simulink model "ctrl_custom_case_c"  (R2016b)
settings: Solver=ode4  StartTime=0.0  StopTime=inf  FixedStep=0.01  RelTol=1e-3  EnableMultiTasking=on
undefined symbols (not defined in the file): alpha1, alpha2, b, C1, C2, center, D, inv_M, M, pd_final, pd_initial, R, Umax_1, Umax_2
libraries: lib x9, simulink x5
(part 3 of 3)

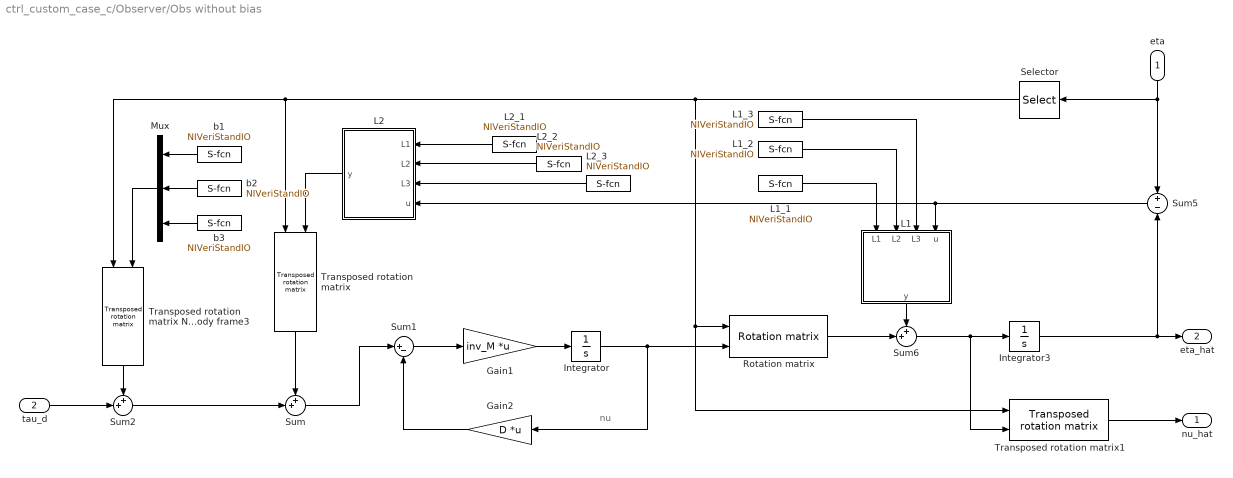
== system ctrl_custom_case_c/Observer/Obs without bias ==
  note: nu
  eta : Inport
  tau_d : Inport  Port=2
  Gain1 : Gain  Gain=inv_M  Multiplication=Matrix(K*u)
  Gain2 : Gain  Gain=D  Multiplication=Matrix(K*u)
  Integrator : Integrator
  Integrator3 : Integrator
  L1 : MATLAB Function  TreatAsAtomicUnit=on
  L1_1 : S-Function  Priority=1  FunctionName=NIVeriStandIO  Parameters=width dtype portnum stime stype btype  SFunctionDeploymentMode=off  EnableBusSupport=off  mask(NI VeriStand Inport){portnum=1, width=-1, stime=-1, dtype=auto, stype=auto, btype=1}
      mask prompts: portnum "Port number:"; width "Port dimensions (-1 for dynamically sized):"; stime "Sample time (-1 for inherited):"; dtype "Data type:"; stype "Signal type:"; btype "Block type:"
      mask help: Use this inport on any level of nested subsystems to allow NI VeriStand software to map signals to it.
      mask init:
      | NIVeriStandIO_init;
      settings: CopyFcn=NIVeriStand_MDL_functions('', 'IO_copy');  DeleteFcn=NIVeriStand_MDL_functions('', 'IO_delete');  MoveFcn=set_param(gcb, 'Mask', 'on');
      mask Callback portnum: NIVeriStand_MDL_functions('', 'IO_setportnum');
      mask TypeOptions dtype: auto | double | single | int8 | uint8 | int16 | uint16 | int32 | uint32 | boolean
      mask Callback dtype: NIVeriStand_MDL_functions('', 'IO_booleansignal');
      mask TypeOptions stype: auto | real | complex
      mask Display:
      | patch([-x x], [-y y], [.90980 .81960 .32156]);
      | plot([xrad -x x xrad], [yrad -y y yrad]);
      | fprintf('NI In%d', portnum);
  L1_2 : S-Function  Priority=2  FunctionName=NIVeriStandIO  Parameters=width dtype portnum stime stype btype  SFunctionDeploymentMode=off  EnableBusSupport=off  mask(NI VeriStand Inport){portnum=2, width=-1, stime=-1, dtype=auto, stype=auto, btype=1}
      mask prompts: portnum "Port number:"; width "Port dimensions (-1 for dynamically sized):"; stime "Sample time (-1 for inherited):"; dtype "Data type:"; stype "Signal type:"; btype "Block type:"
      mask help: Use this inport on any level of nested subsystems to allow NI VeriStand software to map signals to it.
      mask init:
      | NIVeriStandIO_init;
      settings: CopyFcn=NIVeriStand_MDL_functions('', 'IO_copy');  DeleteFcn=NIVeriStand_MDL_functions('', 'IO_delete');  MoveFcn=set_param(gcb, 'Mask', 'on');
      mask Callback portnum: NIVeriStand_MDL_functions('', 'IO_setportnum');
      mask TypeOptions dtype: auto | double | single | int8 | uint8 | int16 | uint16 | int32 | uint32 | boolean
      mask Callback dtype: NIVeriStand_MDL_functions('', 'IO_booleansignal');
      mask TypeOptions stype: auto | real | complex
      mask Display:
      | patch([-x x], [-y y], [.90980 .81960 .32156]);
      | plot([xrad -x x xrad], [yrad -y y yrad]);
      | fprintf('NI In%d', portnum);
  L1_3 : S-Function  Priority=3  FunctionName=NIVeriStandIO  Parameters=width dtype portnum stime stype btype  SFunctionDeploymentMode=off  EnableBusSupport=off  mask(NI VeriStand Inport){portnum=3, width=-1, stime=-1, dtype=auto, stype=auto, btype=1}
      mask prompts: portnum "Port number:"; width "Port dimensions (-1 for dynamically sized):"; stime "Sample time (-1 for inherited):"; dtype "Data type:"; stype "Signal type:"; btype "Block type:"
      mask help: Use this inport on any level of nested subsystems to allow NI VeriStand software to map signals to it.
      mask init:
      | NIVeriStandIO_init;
      settings: CopyFcn=NIVeriStand_MDL_functions('', 'IO_copy');  DeleteFcn=NIVeriStand_MDL_functions('', 'IO_delete');  MoveFcn=set_param(gcb, 'Mask', 'on');
      mask Callback portnum: NIVeriStand_MDL_functions('', 'IO_setportnum');
      mask TypeOptions dtype: auto | double | single | int8 | uint8 | int16 | uint16 | int32 | uint32 | boolean
      mask Callback dtype: NIVeriStand_MDL_functions('', 'IO_booleansignal');
      mask TypeOptions stype: auto | real | complex
      mask Display:
      | patch([-x x], [-y y], [.90980 .81960 .32156]);
      | plot([xrad -x x xrad], [yrad -y y yrad]);
      | fprintf('NI In%d', portnum);
  L2 : MATLAB Function  TreatAsAtomicUnit=on
  L2_1 : S-Function  Priority=4  FunctionName=NIVeriStandIO  Parameters=width dtype portnum stime stype btype  SFunctionDeploymentMode=off  EnableBusSupport=off  mask(NI VeriStand Inport){portnum=4, width=-1, stime=-1, dtype=auto, stype=auto, btype=1}
      mask prompts: portnum "Port number:"; width "Port dimensions (-1 for dynamically sized):"; stime "Sample time (-1 for inherited):"; dtype "Data type:"; stype "Signal type:"; btype "Block type:"
      mask help: Use this inport on any level of nested subsystems to allow NI VeriStand software to map signals to it.
      mask init:
      | NIVeriStandIO_init;
      settings: CopyFcn=NIVeriStand_MDL_functions('', 'IO_copy');  DeleteFcn=NIVeriStand_MDL_functions('', 'IO_delete');  MoveFcn=set_param(gcb, 'Mask', 'on');
      mask Callback portnum: NIVeriStand_MDL_functions('', 'IO_setportnum');
      mask TypeOptions dtype: auto | double | single | int8 | uint8 | int16 | uint16 | int32 | uint32 | boolean
      mask Callback dtype: NIVeriStand_MDL_functions('', 'IO_booleansignal');
      mask TypeOptions stype: auto | real | complex
      mask Display:
      | patch([-x x], [-y y], [.90980 .81960 .32156]);
      | plot([xrad -x x xrad], [yrad -y y yrad]);
      | fprintf('NI In%d', portnum);
  L2_2 : S-Function  Priority=5  FunctionName=NIVeriStandIO  Parameters=width dtype portnum stime stype btype  SFunctionDeploymentMode=off  EnableBusSupport=off  mask(NI VeriStand Inport){portnum=5, width=-1, stime=-1, dtype=auto, stype=auto, btype=1}
      mask prompts: portnum "Port number:"; width "Port dimensions (-1 for dynamically sized):"; stime "Sample time (-1 for inherited):"; dtype "Data type:"; stype "Signal type:"; btype "Block type:"
      mask help: Use this inport on any level of nested subsystems to allow NI VeriStand software to map signals to it.
      mask init:
      | NIVeriStandIO_init;
      settings: CopyFcn=NIVeriStand_MDL_functions('', 'IO_copy');  DeleteFcn=NIVeriStand_MDL_functions('', 'IO_delete');  MoveFcn=set_param(gcb, 'Mask', 'on');
      mask Callback portnum: NIVeriStand_MDL_functions('', 'IO_setportnum');
      mask TypeOptions dtype: auto | double | single | int8 | uint8 | int16 | uint16 | int32 | uint32 | boolean
      mask Callback dtype: NIVeriStand_MDL_functions('', 'IO_booleansignal');
      mask TypeOptions stype: auto | real | complex
      mask Display:
      | patch([-x x], [-y y], [.90980 .81960 .32156]);
      | plot([xrad -x x xrad], [yrad -y y yrad]);
      | fprintf('NI In%d', portnum);
  L2_3 : S-Function  Priority=6  FunctionName=NIVeriStandIO  Parameters=width dtype portnum stime stype btype  SFunctionDeploymentMode=off  EnableBusSupport=off  mask(NI VeriStand Inport){portnum=6, width=-1, stime=-1, dtype=auto, stype=auto, btype=1}
      mask prompts: portnum "Port number:"; width "Port dimensions (-1 for dynamically sized):"; stime "Sample time (-1 for inherited):"; dtype "Data type:"; stype "Signal type:"; btype "Block type:"
      mask help: Use this inport on any level of nested subsystems to allow NI VeriStand software to map signals to it.
      mask init:
      | NIVeriStandIO_init;
      settings: CopyFcn=NIVeriStand_MDL_functions('', 'IO_copy');  DeleteFcn=NIVeriStand_MDL_functions('', 'IO_delete');  MoveFcn=set_param(gcb, 'Mask', 'on');
      mask Callback portnum: NIVeriStand_MDL_functions('', 'IO_setportnum');
      mask TypeOptions dtype: auto | double | single | int8 | uint8 | int16 | uint16 | int32 | uint32 | boolean
      mask Callback dtype: NIVeriStand_MDL_functions('', 'IO_booleansignal');
      mask TypeOptions stype: auto | real | complex
      mask Display:
      | patch([-x x], [-y y], [.90980 .81960 .32156]);
      | plot([xrad -x x xrad], [yrad -y y yrad]);
      | fprintf('NI In%d', portnum);
  Mux : Mux  Inputs=3
  Rotation matrix : lib/Rotation matrix
  Selector : Selector  InputPortWidth=3  IndexOptions=Index vector (dialog)  Indices=[ 3]  OutputSizes=1
  Sum : Sum  Inputs=++|
  Sum1 : Sum  Inputs=|+-
  Sum2 : Sum  Inputs=++|
  Sum5 : Sum  Inputs=+|-
  Sum6 : Sum  Inputs=++|
  Transposed rotation matrix : lib/Transposed rotation matrix
  "Transposed rotation matrix NED -> Body frame3" : lib/Transposed rotation matrix
  Transposed rotation matrix1 : lib/Transposed rotation matrix
  b1 : S-Function  Priority=7  FunctionName=NIVeriStandIO  Parameters=width dtype portnum stime stype btype  SFunctionDeploymentMode=off  EnableBusSupport=off  mask(NI VeriStand Inport){portnum=7, width=-1, stime=-1, dtype=auto, stype=auto, btype=1}
      mask prompts: portnum "Port number:"; width "Port dimensions (-1 for dynamically sized):"; stime "Sample time (-1 for inherited):"; dtype "Data type:"; stype "Signal type:"; btype "Block type:"
      mask help: Use this inport on any level of nested subsystems to allow NI VeriStand software to map signals to it.
      mask init:
      | NIVeriStandIO_init;
      settings: CopyFcn=NIVeriStand_MDL_functions('', 'IO_copy');  DeleteFcn=NIVeriStand_MDL_functions('', 'IO_delete');  MoveFcn=set_param(gcb, 'Mask', 'on');
      mask Callback portnum: NIVeriStand_MDL_functions('', 'IO_setportnum');
      mask TypeOptions dtype: auto | double | single | int8 | uint8 | int16 | uint16 | int32 | uint32 | boolean
      mask Callback dtype: NIVeriStand_MDL_functions('', 'IO_booleansignal');
      mask TypeOptions stype: auto | real | complex
      mask Display:
      | patch([-x x], [-y y], [.90980 .81960 .32156]);
      | plot([xrad -x x xrad], [yrad -y y yrad]);
      | fprintf('NI In%d', portnum);
  b2 : S-Function  Priority=8  FunctionName=NIVeriStandIO  Parameters=width dtype portnum stime stype btype  SFunctionDeploymentMode=off  EnableBusSupport=off  mask(NI VeriStand Inport){portnum=8, width=-1, stime=-1, dtype=auto, stype=auto, btype=1}
      mask prompts: portnum "Port number:"; width "Port dimensions (-1 for dynamically sized):"; stime "Sample time (-1 for inherited):"; dtype "Data type:"; stype "Signal type:"; btype "Block type:"
      mask help: Use this inport on any level of nested subsystems to allow NI VeriStand software to map signals to it.
      mask init:
      | NIVeriStandIO_init;
      settings: CopyFcn=NIVeriStand_MDL_functions('', 'IO_copy');  DeleteFcn=NIVeriStand_MDL_functions('', 'IO_delete');  MoveFcn=set_param(gcb, 'Mask', 'on');
      mask Callback portnum: NIVeriStand_MDL_functions('', 'IO_setportnum');
      mask TypeOptions dtype: auto | double | single | int8 | uint8 | int16 | uint16 | int32 | uint32 | boolean
      mask Callback dtype: NIVeriStand_MDL_functions('', 'IO_booleansignal');
      mask TypeOptions stype: auto | real | complex
      mask Display:
      | patch([-x x], [-y y], [.90980 .81960 .32156]);
      | plot([xrad -x x xrad], [yrad -y y yrad]);
      | fprintf('NI In%d', portnum);
  b3 : S-Function  Priority=9  FunctionName=NIVeriStandIO  Parameters=width dtype portnum stime stype btype  SFunctionDeploymentMode=off  EnableBusSupport=off  mask(NI VeriStand Inport){portnum=9, width=-1, stime=-1, dtype=auto, stype=auto, btype=1}
      mask prompts: portnum "Port number:"; width "Port dimensions (-1 for dynamically sized):"; stime "Sample time (-1 for inherited):"; dtype "Data type:"; stype "Signal type:"; btype "Block type:"
      mask help: Use this inport on any level of nested subsystems to allow NI VeriStand software to map signals to it.
      mask init:
      | NIVeriStandIO_init;
      settings: CopyFcn=NIVeriStand_MDL_functions('', 'IO_copy');  DeleteFcn=NIVeriStand_MDL_functions('', 'IO_delete');  MoveFcn=set_param(gcb, 'Mask', 'on');
      mask Callback portnum: NIVeriStand_MDL_functions('', 'IO_setportnum');
      mask TypeOptions dtype: auto | double | single | int8 | uint8 | int16 | uint16 | int32 | uint32 | boolean
      mask Callback dtype: NIVeriStand_MDL_functions('', 'IO_booleansignal');
      mask TypeOptions stype: auto | real | complex
      mask Display:
      | patch([-x x], [-y y], [.90980 .81960 .32156]);
      | plot([xrad -x x xrad], [yrad -y y yrad]);
      | fprintf('NI In%d', portnum);
  nu_hat : Outport
  eta_hat : Outport  Port=2
  wires:
  Sum/1 -> Sum1/1
  Sum6/1 -> Transposed rotation matrix1/2, Integrator3/1
  Transposed rotation matrix1/1 -> nu_hat/1
  L1/1(y) -> Sum6/1
  Rotation matrix/1 -> Sum6/2
  Sum5/1 -> L1/4(u), L2/4(u)
  Gain1/1 -> Integrator/1
  Integrator3/1 -> Sum5/2, eta_hat/1
  L2/1(y) -> Transposed rotation matrix/2
  Transposed rotation matrix/1 -> Sum/1
  Sum1/1 -> Gain1/1
  eta/1 -> Selector/1, Sum5/1
  Gain2/1 -> Sum1/2
  Integrator/1 -> Gain2/1, Rotation matrix/2
  L1_1/1 -> L1/1(L1)
  L1_2/1 -> L1/2(L2)
  L1_3/1 -> L1/3(L3)
  L2_1/1 -> L2/1(L1)
  L2_2/1 -> L2/2(L2)
  L2_3/1 -> L2/3(L3)
  Selector/1 -> Transposed rotation matrix1/1, Rotation matrix/1, Transposed rotation matrix/1, "Transposed rotation matrix NED -> Body frame3"/1
  Mux/1 -> "Transposed rotation matrix NED -> Body frame3"/2
  b1/1 -> Mux/1
  b2/1 -> Mux/2
  b3/1 -> Mux/3
  tau_d/1 -> Sum2/2
  Sum2/1 -> Sum/2
  "Transposed rotation matrix NED -> Body frame3"/1 -> Sum2/1

== system ctrl_custom_case_c/Thrust Allocation-rec/VSP1 ==
  u_1x : Inport
  u_1y : Inport  Port=2
  Atan2 : Trigonometry  Operator=atan2
  Sqrt : Sqrt  SaturateOnIntegerOverflow=on
  Square : Math  Operator=square  SaturateOnIntegerOverflow=on
  Square1 : Math  Operator=square  SaturateOnIntegerOverflow=on
  Sum : Sum  Inputs=|++
  u_1 : Outport
  Alpha_1 : Outport  Port=2
  wires:
  u_1x/1 -> Atan2/2, Square/1
  u_1y/1 -> Square1/1, Atan2/1
  Square/1 -> Sum/1
  Square1/1 -> Sum/2
  Sum/1 -> Sqrt/1
  Sqrt/1 -> u_1/1
  Atan2/1 -> Alpha_1/1

== system ctrl_custom_case_c/Thrust Allocation-rec/VSP2 ==
  u_2x : Inport
  u_2y : Inport  Port=2
  Atan2 : Trigonometry  Operator=atan2
  Sqrt : Sqrt  SaturateOnIntegerOverflow=on
  Square : Math  Operator=square  SaturateOnIntegerOverflow=on
  Square1 : Math  Operator=square  SaturateOnIntegerOverflow=on
  Sum : Sum  Inputs=|++
  u_2 : Outport
  Alpha_2 : Outport  Port=2
  wires:
  Square/1 -> Sum/1
  Square1/1 -> Sum/2
  Sum/1 -> Sqrt/1
  Sqrt/1 -> u_2/1
  u_2x/1 -> Atan2/2, Square/1
  Atan2/1 -> Alpha_2/1
  u_2y/1 -> Atan2/1, Square1/1

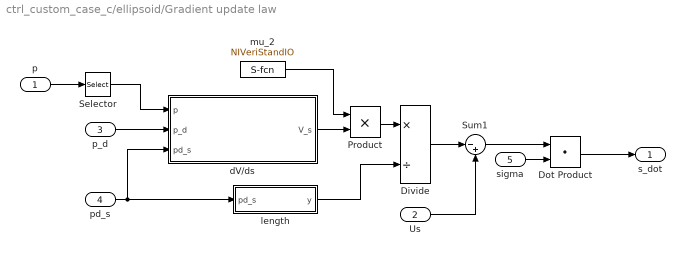
== system ctrl_custom_case_c/ellipsoid/Gradient update law ==
  p : Inport
  Us : Inport  Port=2
  p_d : Inport  Port=3
  pd_s : Inport  Port=4
  sigma : Inport  Port=5
  Divide : Product  Inputs=*/
  Dot Product : DotProduct  InputSameDT=on  OutDataTypeStr=Inherit: Inherit via internal rule
  Product : Product
  Selector : Selector  InputPortWidth=3  IndexOptions=Index vector (dialog)  Indices=[1 2]  OutputSizes=1
  Sum1 : Sum  Inputs=|-+
  "dV/ds  " : MATLAB Function  TreatAsAtomicUnit=on
  length : MATLAB Function  TreatAsAtomicUnit=on
  mu_2 : S-Function  Priority=1  FunctionName=NIVeriStandIO  Parameters=width dtype portnum stime stype btype  SFunctionDeploymentMode=off  EnableBusSupport=off  mask(NI VeriStand Inport){portnum=1, width=-1, stime=-1, dtype=auto, stype=auto, btype=1}
      mask prompts: portnum "Port number:"; width "Port dimensions (-1 for dynamically sized):"; stime "Sample time (-1 for inherited):"; dtype "Data type:"; stype "Signal type:"; btype "Block type:"
      mask help: Use this inport on any level of nested subsystems to allow NI VeriStand software to map signals to it.
      mask init:
      | NIVeriStandIO_init;
      settings: CopyFcn=NIVeriStand_MDL_functions('', 'IO_copy');  DeleteFcn=NIVeriStand_MDL_functions('', 'IO_delete');  MoveFcn=set_param(gcb, 'Mask', 'on');
      mask Callback portnum: NIVeriStand_MDL_functions('', 'IO_setportnum');
      mask TypeOptions dtype: auto | double | single | int8 | uint8 | int16 | uint16 | int32 | uint32 | boolean
      mask Callback dtype: NIVeriStand_MDL_functions('', 'IO_booleansignal');
      mask TypeOptions stype: auto | real | complex
      mask Display:
      | patch([-x x], [-y y], [.90980 .81960 .32156]);
      | plot([xrad -x x xrad], [yrad -y y yrad]);
      | fprintf('NI In%d', portnum);
  s_dot : Outport
  wires:
  Product/1 -> Divide/1
  Divide/1 -> Sum1/1
  "dV/ds  "/1(V_s) -> Product/2
  p_d/1 -> "dV/ds  "/2(p_d)
  pd_s/1 -> "dV/ds  "/3(pd_s), length/1(pd_s)
  length/1(y) -> Divide/2
  Us/1 -> Sum1/2
  Sum1/1 -> Dot Product/1
  Dot Product/1 -> s_dot/1
  sigma/1 -> Dot Product/2
  p/1 -> Selector/1
  Selector/1 -> "dV/ds  "/1(p)
  mu_2/1 -> Product/1

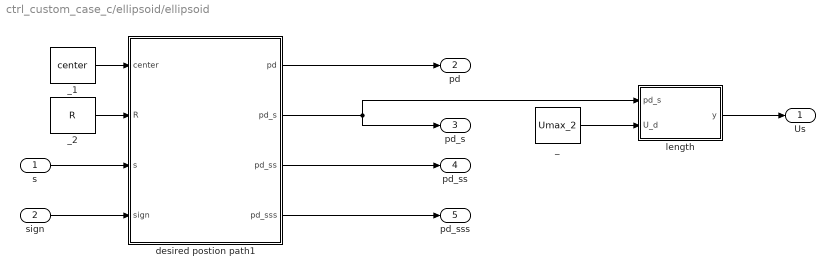
== system ctrl_custom_case_c/ellipsoid/ellipsoid ==
  s : Inport
  sign : Inport  Port=2
  _ : Constant  Value=Umax_2
  _1 : Constant  Value=center
  _2 : Constant  Value=R
  desired postion path1 : MATLAB Function  TreatAsAtomicUnit=on
  length : MATLAB Function  TreatAsAtomicUnit=on
  Us : Outport
  pd : Outport  Port=2
  pd_s : Outport  Port=3
  pd_ss : Outport  Port=4
  pd_sss : Outport  Port=5
  wires:
  _2/1 -> desired postion path1/2(R)
  _1/1 -> desired postion path1/1(center)
  desired postion path1/1(pd) -> pd/1
  desired postion path1/2(pd_s) -> pd_s/1, length/1(pd_s)
  length/1(y) -> Us/1
  s/1 -> desired postion path1/3(s)
  sign/1 -> desired postion path1/4(sign)
  _/1 -> length/2(U_d)
  desired postion path1/3(pd_ss) -> pd_ss/1
  desired postion path1/4(pd_sss) -> pd_sss/1

== system ctrl_custom_case_c/ellipsoid/position controller ==
  p : Inport
  pd : Inport  Port=2
  pd_s : Inport  Port=3
  Us : Inport  Port=4
  K : Gain  Gain=diag([0.1,0.1])  Multiplication=Matrix(K*u)
  Product : Product
  Selector : Selector  InputPortWidth=3  IndexOptions=Index vector (dialog)  Indices=[1 2]  OutputSizes=1
  Sum : Sum  Inputs=|+-
  Sum1 : Sum  Inputs=|-+
  u : Outport
  wires:
  Sum/1 -> K/1
  pd_s/1 -> Product/1
  Us/1 -> Product/2
  K/1 -> Sum1/1
  Product/1 -> Sum1/2
  Sum1/1 -> u/1
  pd/1 -> Sum/2
  p/1 -> Selector/1
  Selector/1 -> Sum/1

== system ctrl_custom_case_c/ellipsoid/switch ==
  s : Inport
  Memory : Memory  X0=1
  switch with respect to s : MATLAB Function  TreatAsAtomicUnit=on
  sign : Outport
  wires:
  switch with respect to s/1(sign_) -> sign/1, Memory/1
  Memory/1 -> switch with respect to s/2(prev_sign)
  s/1 -> switch with respect to s/1(s)

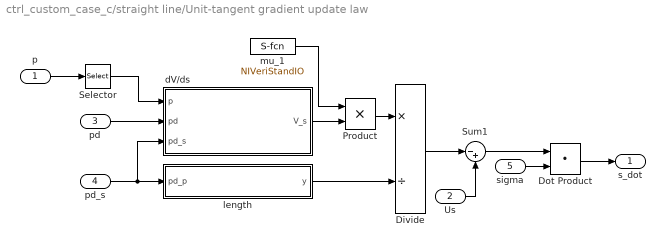
== system ctrl_custom_case_c/straight line/Unit-tangent gradient update law ==
  p : Inport
  Us : Inport  Port=2
  pd : Inport  Port=3
  pd_s : Inport  Port=4
  sigma : Inport  Port=5
  Divide : Product  Inputs=*/
  Dot Product : DotProduct  InputSameDT=on  OutDataTypeStr=Inherit: Inherit via internal rule
  Product : Product
  Selector : Selector  InputPortWidth=3  IndexOptions=Index vector (dialog)  Indices=[1 2]  OutputSizes=1
  Sum1 : Sum  Inputs=|-+
  "dV/ds  " : MATLAB Function  TreatAsAtomicUnit=on
  length : MATLAB Function  TreatAsAtomicUnit=on
  mu_1 : S-Function  Priority=1  FunctionName=NIVeriStandIO  Parameters=width dtype portnum stime stype btype  SFunctionDeploymentMode=off  EnableBusSupport=off  mask(NI VeriStand Inport){portnum=1, width=-1, stime=-1, dtype=auto, stype=auto, btype=1}
      mask prompts: portnum "Port number:"; width "Port dimensions (-1 for dynamically sized):"; stime "Sample time (-1 for inherited):"; dtype "Data type:"; stype "Signal type:"; btype "Block type:"
      mask help: Use this inport on any level of nested subsystems to allow NI VeriStand software to map signals to it.
      mask init:
      | NIVeriStandIO_init;
      settings: CopyFcn=NIVeriStand_MDL_functions('', 'IO_copy');  DeleteFcn=NIVeriStand_MDL_functions('', 'IO_delete');  MoveFcn=set_param(gcb, 'Mask', 'on');
      mask Callback portnum: NIVeriStand_MDL_functions('', 'IO_setportnum');
      mask TypeOptions dtype: auto | double | single | int8 | uint8 | int16 | uint16 | int32 | uint32 | boolean
      mask Callback dtype: NIVeriStand_MDL_functions('', 'IO_booleansignal');
      mask TypeOptions stype: auto | real | complex
      mask Display:
      | patch([-x x], [-y y], [.90980 .81960 .32156]);
      | plot([xrad -x x xrad], [yrad -y y yrad]);
      | fprintf('NI In%d', portnum);
  s_dot : Outport
  wires:
  Product/1 -> Divide/1
  Divide/1 -> Sum1/1
  "dV/ds  "/1(V_s) -> Product/2
  pd/1 -> "dV/ds  "/2(pd)
  pd_s/1 -> "dV/ds  "/3(pd_s), length/1(pd_p)
  length/1(y) -> Divide/2
  Us/1 -> Sum1/2
  Sum1/1 -> Dot Product/1
  Dot Product/1 -> s_dot/1
  sigma/1 -> Dot Product/2
  p/1 -> Selector/1
  Selector/1 -> "dV/ds  "/1(p)
  mu_1/1 -> Product/1

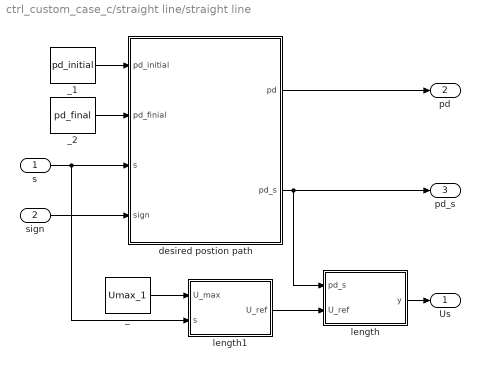
== system ctrl_custom_case_c/straight line/straight line ==
  s : Inport
  sign : Inport  Port=2
  _ : Constant  Value=Umax_1
  _1 : Constant  Value=pd_initial
  _2 : Constant  Value=pd_final
  desired postion path : MATLAB Function  TreatAsAtomicUnit=on
  length : MATLAB Function  TreatAsAtomicUnit=on
  length1 : MATLAB Function  TreatAsAtomicUnit=on
  Us : Outport
  pd : Outport  Port=2
  pd_s : Outport  Port=3
  wires:
  _2/1 -> desired postion path/2(pd_finial)
  _1/1 -> desired postion path/1(pd_initial)
  desired postion path/1(pd) -> pd/1
  desired postion path/2(pd_s) -> length/1(pd_s), pd_s/1
  length/1(y) -> Us/1
  s/1 -> length1/2(s), desired postion path/3(s)
  sign/1 -> desired postion path/4(sign)
  _/1 -> length1/1(U_max)
  length1/1(U_ref) -> length/2(U_ref)

== system ctrl_custom_case_c/straight line/switch ==
  s : Inport
  Memory : Memory  X0=1
  switch with respect to s : MATLAB Function  TreatAsAtomicUnit=on
  sign : Outport
  wires:
  switch with respect to s/1(sign_) -> sign/1, Memory/1
  Memory/1 -> switch with respect to s/2(prev_sign)
  s/1 -> switch with respect to s/1(s)

== matlab function ctrl_custom_case_c/Observer/Obs without bias/L1 ==
  data: L1 input; L2 input; L3 input; u input; y output
function y = fcn(L1,L2,L3,u)

y = diag([L1,L2,L3])*u;

== matlab function ctrl_custom_case_c/MATLAB Function ==
  data: x output; u input; y output
function [x,y] = fcn(u)

x = 1;
y = 0;
if u == 1
    x = 1;
    y = 0;
end

if u == 2
    x = 0;
    y = 1;
end

== matlab function ctrl_custom_case_c/Observer/Obs without bias/L2 ==
  data: L1 input; L2 input; L3 input; u input; y output
function y = fcn(L1,L2,L3,u)

y = diag([L1,L2,L3])*u;

== matlab function ctrl_custom_case_c/Observer/Obs with bias/L1 ==
  data: L1 input; L2 input; L3 input; u input; y output
function y = fcn(L1,L2,L3,u)

y = diag([L1,L2,L3])*u;

== matlab function ctrl_custom_case_c/Observer/Obs with bias/L2 ==
  data: L1 input; L2 input; L3 input; u input; y output
function y = fcn(L1,L2,L3,u)

y = diag([L1,L2,L3])*u;

== matlab function ctrl_custom_case_c/Observer/Obs with bias/L3 ==
  data: L1 input; L2 input; L3 input; u input; y output
function y = fcn(L1,L2,L3,u)

y = diag([L1,L2,L3])*u;

== matlab function ctrl_custom_case_c/Switch_function1 ==
  data: ArrowL input; switch_signal output; ArrowR input; temp input
%% Function that takes in impulse button sigals [0,1] and sends out a 
% different signal depentent pn which button has been pressed

function switch_signal = fcn(ArrowL,ArrowR,temp)
%#codegen
persistent signal;

signal = temp;

if ArrowL ~= 0
    signal = 1;
end

if ArrowR ~= 0
    signal = 2;
end


switch_signal = signal;

== matlab function ctrl_custom_case_c/Switch_function ==
  data: ArrowL input; switch_signal output; ArrowR input; temp input
%% Function that takes in impulse button sigals [0,1] and sends out a 
% different signal depentent pn which button has been pressed

function switch_signal = fcn(ArrowL,ArrowR,temp)
%#codegen
persistent signal;

signal = temp;

if ArrowL ~= 0
    signal = 1;
end

if ArrowR ~= 0
    signal = 2;
end


switch_signal = signal;

== matlab function ctrl_custom_case_c/MATLAB Function1 ==
  data: x output; u input; y output
function [x,y] = fcn(u)

x = 1;
y = 0;
if u == 1
    x = 1;
    y = 0;
end

if u == 2
    x = 0;
    y = 1;
end

== matlab function ctrl_custom_case_c/straight line/Unit-tangent gradient update law/dV//ds   ==
  data: p input; V_s output; pd input; pd_s input
function V_s = fcn(p, pd, pd_s)
e = p - pd;
V_s = - transpose(e)*pd_s;

== matlab function ctrl_custom_case_c/straight line/Unit-tangent gradient update law/length ==
  data: pd_p input; y output
function y = fcn(pd_p)

y = sqrt(pd_p(1)^2 + pd_p(2)^2);

== matlab function ctrl_custom_case_c/straight line/straight line/desired postion path ==
  data: pd_initial input; pd_finial input; pd output; pd_s output; s input size=1; sign input size=1
function [pd,pd_s] = fcn(pd_initial,pd_finial,s, sign)

if s >= 1,
    s = 1;
end

pd_s = [ (pd_finial(1)-pd_initial(1))*sign; 
                (pd_finial(2)-pd_initial(2))*sign];
% |pd_s| = |pd_p|*|s_dot|

pd =  [(pd_finial(1)-pd_initial(1))*s + pd_initial(1);
        (pd_finial(2)-pd_initial(2))*s + pd_initial(2)];   
end

== matlab function ctrl_custom_case_c/straight line/straight line/length ==
  data: pd_s input; y output; U_ref input
function y = fcn(pd_s,U_ref)

y = U_ref/sqrt(pd_s(1)^2 + pd_s(2)^2);

== matlab function ctrl_custom_case_c/straight line/straight line/length1 ==
  data: U_max input; U_ref output; s input
function U_ref = fcn(U_max,s)

if s > 1
    s = 1;
elseif s < 0
    s = 0;
end

U_ref = U_max;

== matlab function ctrl_custom_case_c/straight line/MATLAB Function ==
  data: pd input; pd_s input; eta_d output
function eta_d = fcn(pd,pd_s)
%#codegen
psi_d = atan(pd_s(2)/pd_s(1));

eta_d = [pd(1); pd(2); psi_d];

== matlab function ctrl_custom_case_c/straight line/MATLAB Function1 ==
  data: pd_s input; eta_dot output; s_dot input
function eta_dot = fcn(pd_s, s_dot)
eta_dot = [pd_s(1)*s_dot;pd_s(2)*s_dot;0];

== matlab function ctrl_custom_case_c/ellipsoid/Gradient update law/dV//ds   ==
  data: p input; V_s output; p_d input; pd_s input
function V_s = fcn(p, p_d, pd_s)
V_s = - transpose(p - p_d)*pd_s;

== matlab function ctrl_custom_case_c/ellipsoid/Gradient update law/length ==
  data: pd_s input; y output
function y = fcn(pd_s)

y = sqrt(pd_s(1)^2 + pd_s(2)^2);

== matlab function ctrl_custom_case_c/ellipsoid/MATLAB Function ==
  data: pd input; pd_s input; eta_d output
function eta_d = fcn(pd,pd_s)
%#codegen
psi_d = atan(pd_s(2)/pd_s(1));

eta_d = [pd(1); pd(2); psi_d];

== matlab function ctrl_custom_case_c/ellipsoid/MATLAB Function1 ==
  data: pd_s input; eta_dot output; pd_ss input; s_dot input
function eta_dot = fcn(pd_s, pd_ss, s_dot)
%#codegen
psi_d_dot =(pd_s(1)*pd_ss(2)-pd_s(2)*pd_ss(1))/(pd_s(1)^2+ pd_s(2)^2);
eta_dot = [pd_s(1)*s_dot;pd_s(2)*s_dot;psi_d_dot];

== matlab function ctrl_custom_case_c/Controller_parameters/calculating alpha1 ==
  data: z1 input size=[3 1]; K1 input; alpha1 output; eta_d_dot input size=[3 1]; eta_hat input size=[3 1]
function alpha1 = fcn(z1,K1, eta_d_dot, eta_hat)
%#codegen
psi_hat = eta_hat(3);
R = [   cos(psi_hat)    -sin(psi_hat)   0;
        sin(psi_hat)    cos(psi_hat)    0;
        0           0           0;];  

alpha1 = -K1*z1 + transpose(R)*eta_d_dot;

== matlab function ctrl_custom_case_c/ellipsoid/ellipsoid/length ==
  data: pd_s input; y output; U_d input
function y = fcn(pd_s,U_d)

y = U_d/sqrt(pd_s(1)^2 + pd_s(2)^2);

== matlab function ctrl_custom_case_c/Controller_parameters/calculating alpha1_dot ==
  data: eta_hat input; nu_hat input size=[3 1]; K1 input size=[3 3]; eta_d_dot input size=[3 1]; alpha1_dot output size=[3 1]; z1 input; z2 input; eta_d_dot2 input
function alpha1_dot = fcn(eta_hat, nu_hat, K1, eta_d_dot, z1, z2, eta_d_dot2)
%#codegen
r = [0 0 1]*nu_hat;
S = r*[0 -1 0;
     1 0 0;
     0 0 0;];
psi_hat = eta_hat(3);
R = [   cos(psi_hat)    -sin(psi_hat)   0;
        sin(psi_hat)    cos(psi_hat)    0;
        0           0           0;];  

alpha1_dot = K1*(K1+S)*z1 - K1*z2 - S*transpose(R)*eta_d_dot + transpose(R)*eta_d_dot2;

== matlab function ctrl_custom_case_c/ellipsoid/switch/switch with respect to s ==
  data: s input; sign_ output; prev_sign input
function sign_ = fcn(s, prev_sign)

if s > 1 
    sign_ = -1;
elseif s <= 0
        sign_ = 1;
else
    sign_ = prev_sign;
end

== matlab function ctrl_custom_case_c/ellipsoid/ellipsoid/desired postion path1 ==
  data: center input; R input; pd output; pd_s output; s input size=1; sign input size=1; pd_ss output; pd_sss output
function [pd,pd_s, pd_ss, pd_sss] = fcn(center, R, s, sign)

% if s >= 1,
%     s = 1;
% end

pd_sss = [ 8*pi*pi*pi*R(1)*sin(2*pi*s)*sign;
           -8*pi*pi*pi*R(2)*cos(2*pi*s)*sign];
       
pd_ss = [ -4*pi*pi*R(1)*cos(2*pi*s)*sign;
           -4*pi*pi*R(2)*sin(2*pi*s)*sign];
       
pd_s = [ -2*pi*R(1)*sin(2*pi*s)*sign; 
         2*pi*R(2)*cos(2*pi*s)*sign];

pd =  [R(1)*cos(2*pi*s)+center(1);
         R(2)*sin(2*pi*s)+center(2)];   
end

== matlab function ctrl_custom_case_c/ellipsoid/MATLAB Function2 ==
  data: pd_s input; pd_ss input; eta_dot2 output; pd_sss input; s_dot input
function eta_dot2 = fcn(pd_s, pd_ss, pd_sss,s_dot)
%#codegen
psi_d_dot2 =(pd_s(1)*pd_sss(2)-pd_s(2)*pd_sss(1))/(pd_s(1)^2+ pd_s(2)^2)
             - (pd_s(1)*pd_ss(2)-pd_s(2)*pd_ss(1))*(2*pd_s(1)*pd_ss(1)+2*pd_s(2)*pd_ss(2))/(pd_s(1)^2+ pd_s(2)^2)^2;
eta_dot2 = [pd_ss(1)*s_dot;pd_ss(2)*s_dot;psi_d_dot2];

== matlab function ctrl_custom_case_c/Controller_parameters/calculating z1 in BODY-frame ==
  data: z1 output size=[3 1]; eta_hat input size=[3 1]; eta_d input size=[3 1]
function z1 = fcn(eta_hat, eta_d)
%#codegen
psi_hat = eta_hat(3);
R = [   cos(psi_hat)    -sin(psi_hat)   0;
        sin(psi_hat)    cos(psi_hat)    0;
        0           0           0;];  
z1 = transpose(R)*(eta_hat-eta_d);

== matlab function ctrl_custom_case_c/Controller_parameters/calculating z2 ==
  data: z2 output size=[3 1]; nu input size=[3 1]; alpha1 input size=[3 1]
function z2 = fcn(nu, alpha1)
%#codegen

z2 = nu-alpha1;

== matlab function ctrl_custom_case_c/MATLAB Function2 ==
  data: eta_hat input; tau_d output; M input; D input; b input; z1 input; z2 input; alpha1_s input; alpha1 input; K2 input
function tau_d = fcn(eta_hat, M, D, b, z1, z2, alpha1_s, alpha1, K2)
%#codegen
psi_hat = eta_hat(3);
R = [   cos(psi_hat)    -sin(psi_hat)   0;
        sin(psi_hat)    cos(psi_hat)    0;
        0           0           0;];  
tau_d = -z1 + D*alpha1 - transpose(R)*b + M*alpha1_s - K2*z2;

== matlab function ctrl_custom_case_c/straight line/switch/switch with respect to s ==
  data: s input; sign_ output; prev_sign input
function sign_ = fcn(s, prev_sign)

if s > 1 
    sign_ = -1;
elseif s <= 0
        sign_ = 1;
else
    sign_ = prev_sign;
end

== matlab function ctrl_custom_case_c/L3 ==
  data: L1 input; L2 input; L3 input; y output
function y = fcn(L1,L2,L3)

y = diag([L1,L2,L3]);

== matlab function ctrl_custom_case_c/L1 ==
  data: L1 input; L2 input; L3 input; y output
function y = fcn(L1,L2,L3)

y = diag([L1,L2,L3]);
